simulink model "FM"  (R2014b)
settings: Solver=ode45  StartTime=0.0  StopTime=10.0  RelTol=1e-3
libraries: commanapbnd3 x2, dsparch4 x1, commnoisgen2 x1, dspsrcs4 x1
settings Model: Creator=TY  LastModifiedBy=TY

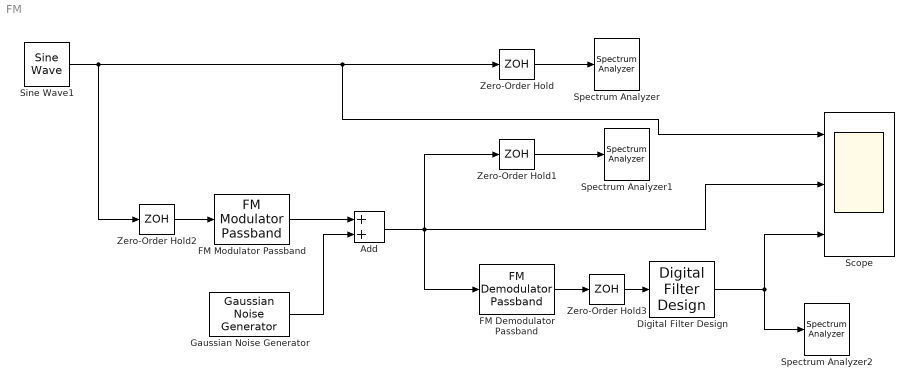
== system FM ==
  Add : Sum
  Digital Filter Design : dsparch4/Digital Filter Design  mwdsp_browser_bugfix_var=off
  FM Demodulator Passband : commanapbnd3/FM Demodulator Passband  Fc=300  Ph=0  Kc=100  Ho=200
  FM Modulator Passband : commanapbnd3/FM Modulator Passband  Fc=300  Ph=0  Kc=150
  Gaussian Noise Generator : commnoisgen2/Gaussian Noise Generator  m=0  d=0  s=41  Ts=1/1000  frameBased=off  sampPerFrame=1  orient=off  outDataType=double
  Scope : Scope  NumInputPorts=3
      settings: YMin=-5~-5~-5  YMax=5~5~5
  Sine Wave1 : dspsrcs4/Sine Wave  Amplitude=1  Frequency=9  Phase=pi  SampleMode=Discrete  OutComplex=Real  CompMethod=Trigonometric fcn  TableSize=Speed  SampleTime=1/10000  SamplesPerFrame=1  ResetState=Restart at time zero  dataType=double  wordLen=16  udDataType=sfix(16)  fracBitsMode=Best precision  numFracBits=15  OutDataTypeStr=double  LastOutDataTypeStr=double
  Spectrum Analyzer : SpectrumAnalyzer
  Spectrum Analyzer1 : SpectrumAnalyzer
  Spectrum Analyzer2 : SpectrumAnalyzer
  Zero-Order Hold : ZeroOrderHold  SampleTime=1/500
  Zero-Order Hold1 : ZeroOrderHold  SampleTime=1/1000
  Zero-Order Hold2 : ZeroOrderHold  SampleTime=1/10000
  Zero-Order Hold3 : ZeroOrderHold  SampleTime=1/500
  wires:
  Zero-Order Hold/1 -> Spectrum Analyzer/1
  Zero-Order Hold1/1 -> Spectrum Analyzer1/1
  Zero-Order Hold2/1 -> FM Modulator Passband/1
  Sine Wave1/1 -> Zero-Order Hold2/1, Zero-Order Hold/1, Scope/1
  FM Demodulator Passband/1 -> Zero-Order Hold3/1
  Digital Filter Design/1 -> Scope/3, Spectrum Analyzer2/1
  Zero-Order Hold3/1 -> Digital Filter Design/1
  Gaussian Noise Generator/1 -> Add/2
  FM Modulator Passband/1 -> Add/1
  Add/1 -> FM Demodulator Passband/1, Scope/2, Zero-Order Hold1/1
